simulink model "carcontrol"  (R2022b)
settings: Solver=FixedStepAuto  StartTime=0.0  StopTime=10.0  RelTol=1e-3  EnableMultiTasking=on
libraries: arduinolib x10, simulink x10, arduinosensorlib x1
settings Model: ExtModeTrigDuration=2  Creator=baris  LastModifiedBy=baris
settings OptimizationCC: EnhancedBackFolding=on  PassReuseOutputArgsAs=Individual arguments  ZeroExternalMemoryAtStartup=off  ZeroInternalMemoryAtStartup=off  MaxStackSize=64  OptimizeBlockOrder=speed  DifferentSizesBufferReuse=on  OptimizationCustomize=off  EfficientTunableParamExpr=on
settings DebuggingCC: ParameterTunabilityLossMsg=error
settings HardwareCC: ProdBitPerInt=16  ProdBitPerPointer=16  ProdBitPerSizeT=16  ProdBitPerPtrDiffT=16  ProdLargestAtomicFloat=None  ProdWordSize=8  ProdHWDeviceType=Atmel->AVR  UseEmbeddedCoderFeatures=off  UseSimulinkCoderFeatures=off
settings SFSimCC: MATLABDynamicMemAlloc=off
settings RTWCC: Description=Embedded Coder  SystemTargetFile=ert.tlc  HardwareBoard=Arduino Uno  TLCOptions=-aInlineSetEventsForThisBaseRateFcn=TLC_FALSE -aSuppressMultiTaskScheduler=TLC_FALSE -aRateBasedStepFcn=1  TemplateMakefile=ert_default_tmf  Toolchain=Arduino AVR  BuildConfiguration=Faster Runs
settings CodeAppCC: ForceParamTrailComments=on  IgnoreCustomStorageClasses=off  OperatorAnnotations=on  SimulinkDataObjDesc=on  SFDataObjDesc=on  MangleLength=10  InsertBlockDesc=on
settings ERTTargetCC: SupportContinuousTime=on  SupportNonInlinedSFcns=on  SupportVariableSizeSignals=on  ExtModeTransport=3  ExtModeStaticAlloc=on  ExtModeAutomaticAllocSize=off  ExtModeStaticAllocSize=250  ExtModeMexFile=ext_xcp  ExtModeIntrfLevel=Level2 - Open

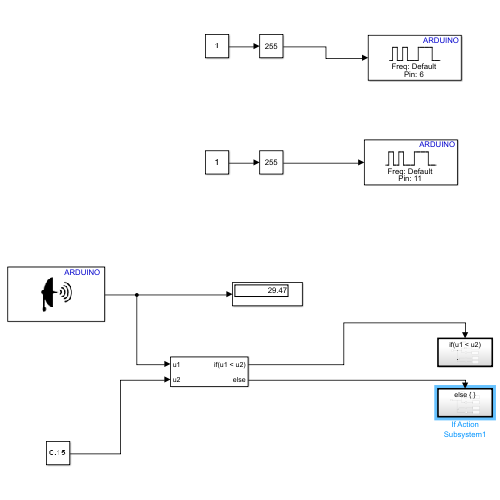
[thumbnail: Simulink's stored preview of the top-level diagram]
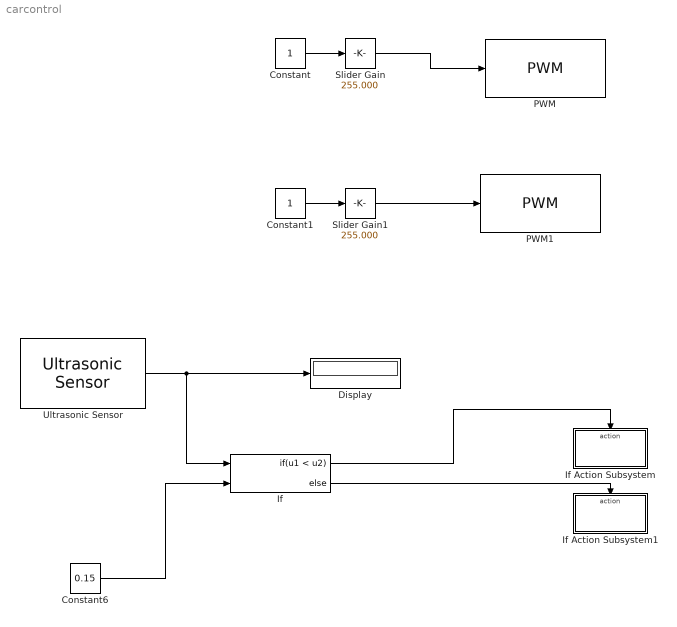
== system carcontrol ==
  Constant : Constant
  Constant1 : Constant
  Constant6 : Constant  Value=0.15
  Display : Display
  If : If  NumInputs=2  IfExpression=u1 < u2
  If Action Subsystem : Subsystem  TreatAsAtomicUnit=on
  If Action Subsystem1 : Subsystem  TreatAsAtomicUnit=on
  PWM : arduinolib/PWM  pinNumber=6  frequencyType=Default  desiredFrequency=490.2  achievableFrequency=490.2
  PWM1 : arduinolib/PWM  pinNumber=11  frequencyType=Default  desiredFrequency=490.2  achievableFrequency=490.2
  Slider Gain : simulink/Math Operations/Slider Gain  gain=255.000  low=0  high=255
  Slider Gain1 : simulink/Math Operations/Slider Gain  gain=255.000  low=0  high=255
  Ultrasonic Sensor : arduinosensorlib/Ultrasonic Sensor  NumSignalPins=2  TrigPin=3  EchoPin=2  SignalPin=3  SampleTime_=0.1  blockPlatform=ARDUINO
  wires:
  Constant/1 -> Slider Gain/1
  Slider Gain1/1 -> PWM1/1
  Constant1/1 -> Slider Gain1/1
  Slider Gain/1 -> PWM/1
  Ultrasonic Sensor/1 -> If/1, Display/1
  Constant6/1 -> If/2
  If/2 -> If Action Subsystem1/Action
  If/1 -> If Action Subsystem/Action

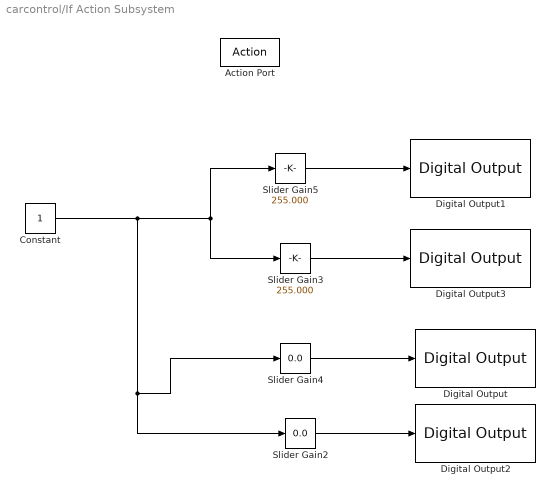
== system carcontrol/If Action Subsystem ==
  Action Port : ActionPort  ActionPortLabel=if(u1 < u2)
  Constant : Constant
  Digital Output : arduinolib/Digital Output  pinNumber=9  Direction=output  blockPlatform=arduino
  Digital Output1 : arduinolib/Digital Output  pinNumber=10  Direction=output  blockPlatform=arduino
  Digital Output2 : arduinolib/Digital Output  pinNumber=8  Direction=output  blockPlatform=arduino
  Digital Output3 : arduinolib/Digital Output  pinNumber=7  Direction=output  blockPlatform=arduino
  Slider Gain2 : simulink/Math Operations/Slider Gain  gain=0.0  low=0  high=255
  Slider Gain3 : simulink/Math Operations/Slider Gain  gain=255.000  low=0  high=255
  Slider Gain4 : simulink/Math Operations/Slider Gain  gain=0.0  low=0  high=255
  Slider Gain5 : simulink/Math Operations/Slider Gain  gain=255.000  low=0  high=255
  wires:
  Slider Gain2/1 -> Digital Output2/1
  Slider Gain3/1 -> Digital Output3/1
  Slider Gain4/1 -> Digital Output/1
  Constant/1 -> Slider Gain2/1, Slider Gain4/1, Slider Gain5/1, Slider Gain3/1
  Slider Gain5/1 -> Digital Output1/1

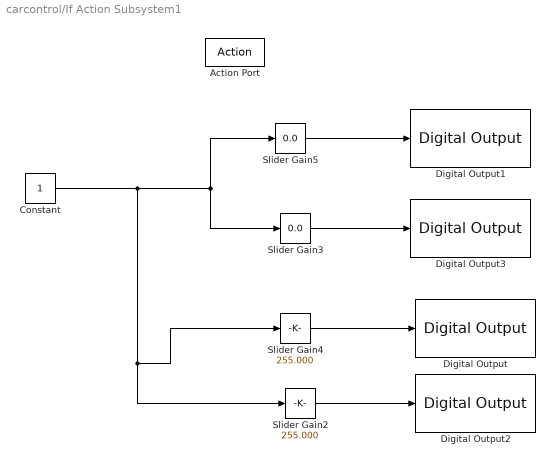
== system carcontrol/If Action Subsystem1 ==
  Action Port : ActionPort  ActionPortLabel=else
  Constant : Constant
  Digital Output : arduinolib/Digital Output  pinNumber=9  Direction=output  blockPlatform=arduino
  Digital Output1 : arduinolib/Digital Output  pinNumber=10  Direction=output  blockPlatform=arduino
  Digital Output2 : arduinolib/Digital Output  pinNumber=8  Direction=output  blockPlatform=arduino
  Digital Output3 : arduinolib/Digital Output  pinNumber=7  Direction=output  blockPlatform=arduino
  Slider Gain2 : simulink/Math Operations/Slider Gain  gain=255.000  low=0  high=255
  Slider Gain3 : simulink/Math Operations/Slider Gain  gain=0.0  low=0  high=255
  Slider Gain4 : simulink/Math Operations/Slider Gain  gain=255.000  low=0  high=255
  Slider Gain5 : simulink/Math Operations/Slider Gain  gain=0.0  low=0  high=255
  wires:
  Constant/1 -> Slider Gain2/1, Slider Gain4/1, Slider Gain5/1, Slider Gain3/1
  Slider Gain5/1 -> Digital Output1/1
  Slider Gain3/1 -> Digital Output3/1
  Slider Gain4/1 -> Digital Output/1
  Slider Gain2/1 -> Digital Output2/1
